simulink model "barcatet_slow_FaraFata"  (R2021a)
settings: Solver=ode8  StartTime=0.0  StopTime=inf  FixedStep=0.1  RelTol=1e-3
libraries: simulink x5, arduinolib x3, arduinosensorlib x3
settings Model: SILPILModeSetting=veronly  ExtModeTrigDuration=2  Creator=CANDRONE  LastModifiedBy=Aspire 5
settings OptimizationCC: EnhancedBackFolding=on  PassReuseOutputArgsAs=Individual arguments  ZeroExternalMemoryAtStartup=off  ZeroInternalMemoryAtStartup=off  MaxStackSize=64  OptimizeBlockOrder=speed  DifferentSizesBufferReuse=on  OptimizationCustomize=off  EfficientTunableParamExpr=on
settings DebuggingCC: ParameterTunabilityLossMsg=error
settings HardwareCC: ProdBitPerInt=16  ProdBitPerPointer=16  ProdBitPerSizeT=16  ProdBitPerPtrDiffT=16  ProdLargestAtomicFloat=None  ProdWordSize=8  ProdHWDeviceType=Atmel->AVR
settings SFSimCC: MATLABDynamicMemAlloc=off
settings RTWCC: SystemTargetFile=ert.tlc  HardwareBoard=Arduino Mega 2560  TemplateMakefile=ert_default_tmf  Toolchain=Arduino AVR
settings CodeAppCC: ForceParamTrailComments=on  IgnoreCustomStorageClasses=off  OperatorAnnotations=on  SimulinkDataObjDesc=on  SFDataObjDesc=on  InsertBlockDesc=on
settings ERTTargetCC: SupportContinuousTime=on  SupportVariableSizeSignals=on  ExtModeStaticAllocSize=2048

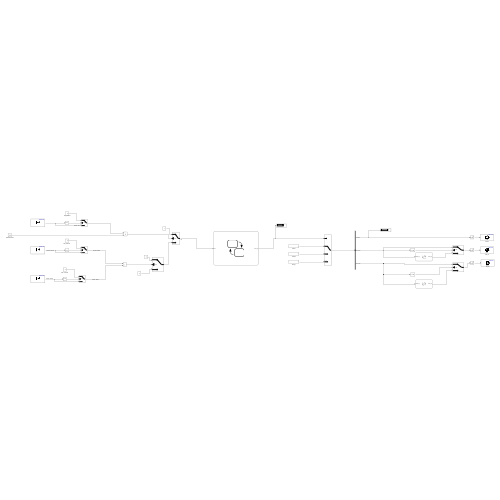
[thumbnail: Simulink's stored preview of the top-level diagram]
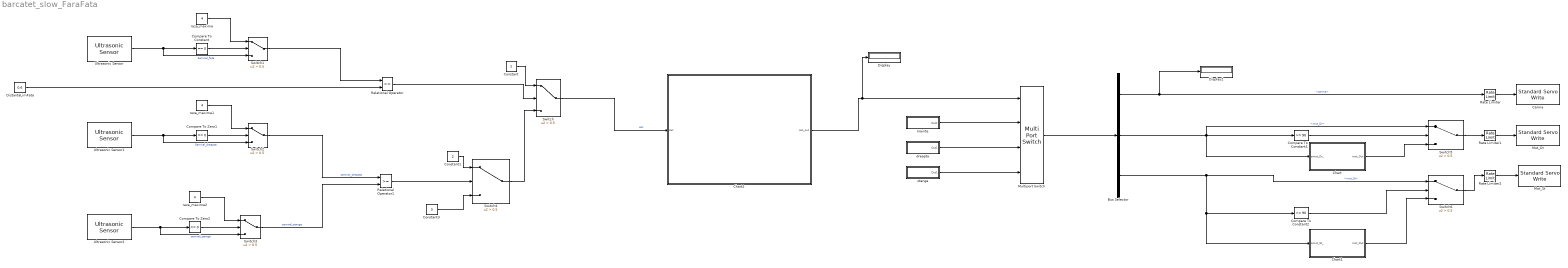
== system barcatet_slow_FaraFata ==
  Bus Selector : BusSelector  OutputSignals=carma,mot_Dr,mot_St
  Carma : arduinolib/Standard Servo Write  pinNumber=3  ServoIndex=0  blockPlatform=ARDUINO
  Chart : Stateflow chart  TreatAsAtomicUnit=on
  Chart1 : Stateflow chart  TreatAsAtomicUnit=on
  Chart2 : Stateflow chart  TreatAsAtomicUnit=on
      settings: PortSchema="{\"entries\":[{\"content\":{\"sides\":[{\"content\":{\"connectorIds\":[]},\"type\":\"ConnectorPlacement.EquallySpacedRectSide\",\"uuid\":\"b65892ab-a4a5-42cf-9574-b562b3ab09c8\"},{\"content\":{\"connectorIds\":[],\"side\":\"RIGHT\"},\"type\":\"ConnectorPlacement.EquallySpacedRectSide\",\"uuid\":\"2dcb0f11-f557-44d4-b00c-5c1b46d969f3\"},{\"content\":{\"connectorIds\":[\"In1\"],\"side\":\"TOP\"},\"type\":\"ConnectorPlacement.EquallySpacedRectSide\",\"uuid\":\"90dfae61-e3ee-4f1a-8a1b-e6404f475ac4\"},{\"content\":{\"connectorIds\":[\"Out1\"],\"side\":\"BOTTOM\"},\"type\":\"ConnectorPlacement.EquallySpacedRectSide\",\"uuid\":\"1ae09705-4430-49f5-b771-2622bfcf56ac\"}]},\"type\":\"ConnectorPlacement.EquallySpacedConnector\",\"uuid\":\"e4b1cea4-b3a8-4687-a2b3-29b89c5ba45a\"}],\"packageUris\":[\"http://schema.mathworks.com/mf0/Connector/R2020b\"],\"version\":\"1.0\"}"
  Compare To Constant : simulink/Logic and Bit Operations/Compare To Constant  relop===  const=0  OutDataTypeStr=boolean
  Compare To Constant1 : simulink/Logic and Bit Operations/Compare To Constant  relop=>=  const=90  OutDataTypeStr=boolean
  Compare To Constant2 : simulink/Logic and Bit Operations/Compare To Constant  relop=>=  const=90  OutDataTypeStr=boolean
  Compare To Zero1 : simulink/Logic and Bit Operations/Compare To Zero  relop===  OutDataTypeStr=boolean
  Compare To Zero2 : simulink/Logic and Bit Operations/Compare To Zero  relop===  OutDataTypeStr=boolean
  Constant : Constant  OutDataTypeStr=double
  Constant1 : Constant  Value=2
  Constant3 : Constant  Value=3
  Display : Display
  Display2 : Display
  DistantaLimFata : Constant  Value=0.6
  Inainte : Subsystem
  Mot_Dr : arduinolib/Standard Servo Write  pinNumber=5  ServoIndex=1  blockPlatform=ARDUINO
  Mot_St : arduinolib/Standard Servo Write  pinNumber=4  ServoIndex=2  blockPlatform=ARDUINO
  Multiport Switch : MultiPortSwitch  DiagnosticForDefault=None
  Rate Limiter : RateLimiter  RisingSlewLimit=5000  FallingSlewLimit=-5000  SampleTimeMode=inherited
  Rate Limiter1 : RateLimiter  RisingSlewLimit=250  FallingSlewLimit=-250  SampleTimeMode=inherited
  Rate Limiter2 : RateLimiter  RisingSlewLimit=250  FallingSlewLimit=-250  SampleTimeMode=inherited
  Relational Operator : RelationalOperator  OutDataTypeStr=boolean  RndMeth=Simplest
  Relational Operator1 : RelationalOperator  OutDataTypeStr=boolean  RndMeth=Simplest
  Switch : Switch  Criteria=u2 > Threshold  Threshold=0.5  OutDataTypeStr=double
  Switch{1..3,5..6} (5 alike) : Switch  Criteria=u2 > Threshold  Threshold=0.5
  Switch4 : Switch  Criteria=u2 > Threshold  Threshold=0.5  OutDataTypeStr=double
  Ultrasonic Sensor : arduinosensorlib/Ultrasonic Sensor  NumSignalPins=2  TrigPin=6  EchoPin=12  SignalPin=3  SampleTime_=0.1  blockPlatform=ARDUINO
      settings: SourceProductBaseCode=ARDUINO
  Ultrasonic Sensor1 : arduinosensorlib/Ultrasonic Sensor  NumSignalPins=2  TrigPin=10  EchoPin=2  SignalPin=3  SampleTime_=0.1  blockPlatform=ARDUINO
      settings: SourceProductBaseCode=ARDUINO
  Ultrasonic Sensor2 : arduinosensorlib/Ultrasonic Sensor  NumSignalPins=2  TrigPin=11  EchoPin=9  SignalPin=3  SampleTime_=0.1  blockPlatform=ARDUINO
      settings: SourceProductBaseCode=ARDUINO
  dreapta : Subsystem
  raza_maxima : Constant  Value=4
  raza_maxima1 : Constant  Value=4
  raza_maxima2 : Constant  Value=4
  stanga : Subsystem
  wires:
  Relational Operator/1 -> Switch/2
  DistantaLimFata/1 -> Relational Operator/2
  Bus Selector/1 -> Display2/1, Rate Limiter/1  "<carma>"
  Bus Selector/2 -> Chart/1(amot_Dr_), Switch5/1, Compare To Constant1/1  "<mot_Dr>"
  Constant/1 -> Switch/1
  Ultrasonic Sensor1/1 -> Switch2/3, Compare To Zero1/1  "Semnal_dreapta"
  Compare To Zero1/1 -> Switch2/2
  Ultrasonic Sensor/1 -> Switch1/3, Compare To Constant/1  "Semnal_fata"
  Compare To Constant/1 -> Switch1/2
  raza_maxima/1 -> Switch1/1
  Switch1/1 -> Relational Operator/1
  raza_maxima1/1 -> Switch2/1
  Ultrasonic Sensor2/1 -> Switch3/3, Compare To Zero2/1  "semnal_stanga"
  raza_maxima2/1 -> Switch3/1
  Compare To Zero2/1 -> Switch3/2
  Switch2/1 -> Relational Operator1/1  "semnal_dreapta"
  Switch3/1 -> Relational Operator1/2  "semnal_stanga"
  Relational Operator1/1 -> Switch4/2
  Constant1/1 -> Switch4/1
  Switch4/1 -> Switch/3
  Rate Limiter/1 -> Carma/1
  Rate Limiter1/1 -> Mot_Dr/1
  Rate Limiter2/1 -> Mot_St/1
  Bus Selector/3 -> Chart1/1(amot_St_), Compare To Constant2/1, Switch6/1  "<mot_St>"
  Compare To Constant1/1 -> Switch5/2
  Switch5/1 -> Rate Limiter1/1
  Chart/1(mot_Out) -> Switch5/3
  Compare To Constant2/1 -> Switch6/2
  Switch6/1 -> Rate Limiter2/1
  Chart1/1(mot_Out) -> Switch6/3
  Constant3/1 -> Switch4/3
  Switch/1 -> Chart2/1(caz)  "caz"
  Multiport Switch/1 -> Bus Selector/1
  Inainte/1(Out1) -> Multiport Switch/2
  Chart2/1(caz_out) -> Display/1, Multiport Switch/1
  dreapta/1(Out1) -> Multiport Switch/3
  stanga/1(Out1) -> Multiport Switch/4

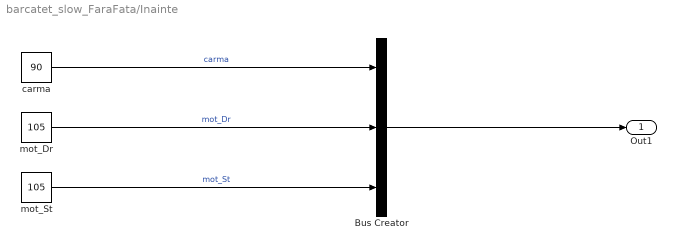
== system barcatet_slow_FaraFata/Inainte ==
  Bus Creator : BusCreator  Inputs=3
  carma : Constant  Value=90
  mot_Dr : Constant  Value=105
  mot_St : Constant  Value=105
  Out1 : Outport
  wires:
  mot_Dr/1 -> Bus Creator/2  "mot_Dr"
  mot_St/1 -> Bus Creator/3  "mot_St"
  carma/1 -> Bus Creator/1  "carma"
  Bus Creator/1 -> Out1/1

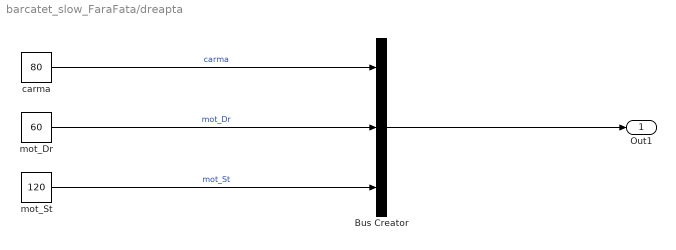
== system barcatet_slow_FaraFata/dreapta ==
  Bus Creator : BusCreator  Inputs=3
  carma : Constant  Value=80
  mot_Dr : Constant  Value=60
  mot_St : Constant  Value=120
  Out1 : Outport
  wires:
  Bus Creator/1 -> Out1/1
  carma/1 -> Bus Creator/1  "carma"
  mot_St/1 -> Bus Creator/3  "mot_St"
  mot_Dr/1 -> Bus Creator/2  "mot_Dr"

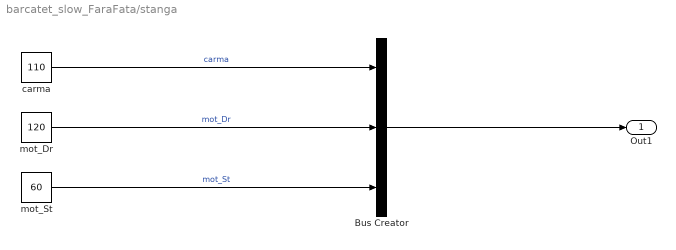
== system barcatet_slow_FaraFata/stanga ==
  Bus Creator : BusCreator  Inputs=3
  carma : Constant  Value=110
  mot_Dr : Constant  Value=120
  mot_St : Constant  Value=60
  Out1 : Outport
  wires:
  mot_Dr/1 -> Bus Creator/2  "mot_Dr"
  mot_St/1 -> Bus Creator/3  "mot_St"
  carma/1 -> Bus Creator/1  "carma"
  Bus Creator/1 -> Out1/1

== stateflow chart barcatet_slow_FaraFata/Chart1 ==
  state reverse_2
    mot_Out = 60;
  state reverse_1
    mot_Out = 90;
  state Reverse_e_activ
    entry:
    mot_Out = 90;
  state reverse_3
    mot_Out = 60;
  reverse_2 -> Reverse_e_activ : [amot_St_ >= 90]
  reverse_1 -> reverse_2 : [after(200,msec)]
  (default) -> Reverse_e_activ
  reverse_3 -> reverse_1 : after(200,msec)
  Reverse_e_activ -> reverse_3 : [amot_St_ < 90]
  data: mot_Out output; amot_St_ input

== stateflow chart barcatet_slow_FaraFata/Chart2 ==
  state default1
    entry:
    caz_out = caz;
    caz_intern = caz;
  state default
    entry:
    caz_out = caz;
    caz_intern = caz;
  state default2
    entry:
    caz_out = caz_intern;
  (default) -> default
  default -> (junction 12) : [hasChanged(caz)]
  (junction 12) -> default1 [order 2] : [caz ==2 || caz == 3]
  (junction 12) -> default [order 1] : [caz ==1]
  default1 -> default2 : [after(10,msec)]
  default2 -> default : [after(0.5,sec)]
  data: caz input double; caz_out output double; caz_intern local

== stateflow chart barcatet_slow_FaraFata/Chart ==
  state reverse_2
    mot_Out = 60;
  state reverse_1
    mot_Out = 90;
  state Reverse_e_activ
    entry:
    mot_Out = 90;
  state reverse_3
    mot_Out = 60;
  reverse_2 -> Reverse_e_activ : [amot_Dr_ >= 90]
  reverse_1 -> reverse_2 : [after(200,msec)]
  (default) -> Reverse_e_activ
  reverse_3 -> reverse_1 : after(200,msec)
  Reverse_e_activ -> reverse_3 : [amot_Dr_ < 90]
  data: mot_Out output; amot_Dr_ input
